simulink subsystem "Ss_controller_nominal_tracking"  (R2024b)
settings: Solver=VariableStepAuto  StartTime=0.0  StopTime=10.0  RelTol=1e-3
values from neighbouring files (symbols this model uses):
  K_stateFB = place(A_c, B_c, p)    [Controller_StateSpace_Lab1.m]
  Nu = Sol(3, :)    [Controller_StateSpace_Lab1.m]
  Nx = Sol(1:2, :)    [Controller_StateSpace_Lab1.m]
undefined symbols (not defined in the file or in its folder): rpm2rads
settings Model: Creator=Utente  LastModifiedBy=Buton

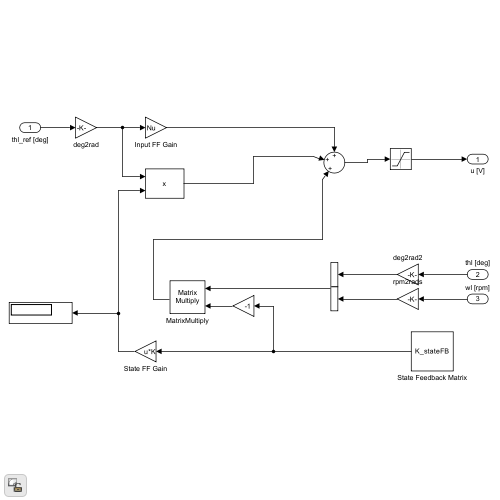
[thumbnail: Simulink's stored preview of the top-level diagram]
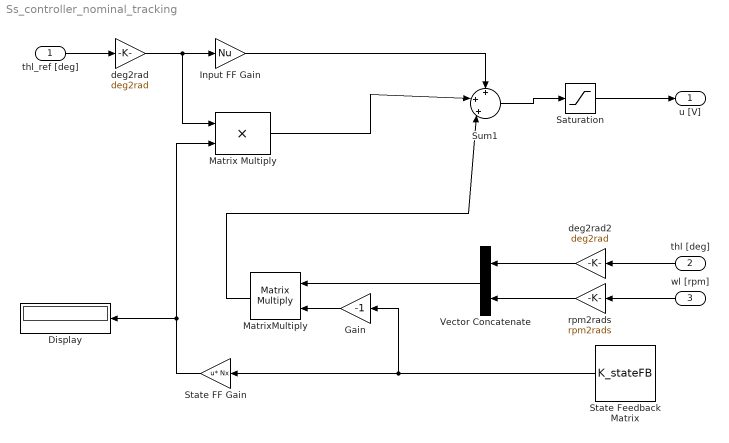
== system Ss_controller_nominal_tracking ==
  thl_ref [deg] : Inport
  thl [deg] : Inport  Port=2
  wl [rpm] : Inport  Port=3
  Display : Display
  Gain : Gain  Gain=-1
  Input FF Gain : Gain  Gain=Nu
  Matrix Multiply : Product
  MatrixMultiply : Product  Multiplication=Matrix(*)
  Saturation : Saturate  UpperLimit=12  LowerLimit=-12
  State FF Gain : Gain  Gain=Nx  Multiplication=Matrix(u*K)
  State Feedback Matrix : Constant  Value=K_stateFB
  Sum1 : Sum  Inputs=+|+|+|
  Vector Concatenate : Concatenate
  deg2rad : Gain  Gain=deg2rad
  deg2rad2 : Gain  Gain=deg2rad
  rpm2rads : Gain  Gain=rpm2rads
  u [V] : Outport
  wires:
  thl [deg]/1 -> deg2rad2/1
  wl [rpm]/1 -> rpm2rads/1
  Sum1/1 -> Saturation/1
  thl_ref [deg]/1 -> deg2rad/1
  deg2rad2/1 -> Vector Concatenate/1
  Saturation/1 -> u [V]/1
  deg2rad/1 -> Input FF Gain/1, Matrix Multiply/1
  Input FF Gain/1 -> Sum1/1
  rpm2rads/1 -> Vector Concatenate/2
  State Feedback Matrix/1 -> State FF Gain/1, Gain/1
  State FF Gain/1 -> Matrix Multiply/2, Display/1
  Matrix Multiply/1 -> Sum1/2
  Gain/1 -> MatrixMultiply/2
  Vector Concatenate/1 -> MatrixMultiply/1
  MatrixMultiply/1 -> Sum1/3
